simulink model "feed_lin_double_deriv_complete"  (R2022b)
settings: Solver=VariableStepAuto  StartTime=0.0  StopTime=15  RelTol=1e-3
model workspace (MAT data in the model file):
  initial_conditions = [0 0 0]
values from neighbouring files (symbols this model uses):
  initial_conditions_1 = [8, 8, 0]    [init.m]
  initial_conditions_2 = [6, 3, 2*pi]    [init.m]
  initial_conditions_3 = [-8, -8, 3*pi/2]    [init.m]
  initial_conditions_trans_2 = state_transformation([0,0,0], initial_conditions_2)    [init.m]
  initial_conditions_trans_3 = state_transformation([0,0,0], initial_conditions_3)    [init.m]
undefined symbols (not defined in the file or in its folder): initial_conditions_trans
settings Model: Creator=dipietrant  LastModifiedBy=Edp
settings SolverCC: AlgebraicLoopSolver=TrustRegion
settings DataIOCC: ReturnWorkspaceOutputs=off
settings DebuggingCC: UnconnectedInputMsg=warning  UnconnectedOutputMsg=warning  UnconnectedLineMsg=warning  SFMachineParentedDataDiag=warning
settings ModelReferenceCC: EnableRefExpFcnMdlSchedulingChecks=on
settings RTWCC: DLArmComputeVersion=19.05

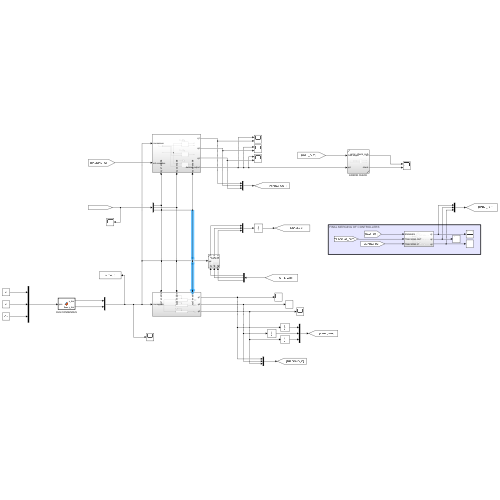
[thumbnail: Simulink's stored preview of the top-level diagram]
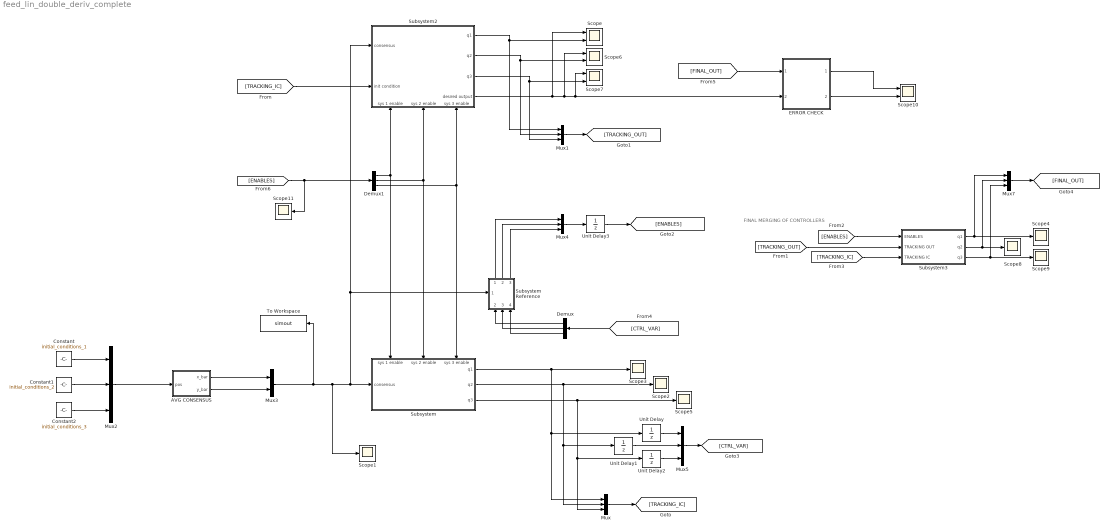
== system feed_lin_double_deriv_complete ==
  note: FINAL MERGING OF CONTROLLERS
  AVG CONSENSUS : MATLAB Function  TreatAsAtomicUnit=on
  Constant : Constant  Value=initial_conditions_1
  Constant1 : Constant  Value=initial_conditions_2
  Constant2 : Constant  Value=initial_conditions_3
  Demux : Demux  Outputs=3
  Demux1 : Demux  Outputs=3
  ERROR CHECK : Subsystem  ReferencedSubsystem=error_check_sub
  Mux{,1..2,4..5,7} (6 alike) : Mux  Inputs=3
  Mux3 : Mux  Inputs=2
  Scope{,6..7,10} (4 alike) : Scope  NumInputPorts=2
  Scope{1..5,8..9,11} (8 alike) : Scope
  Subsystem : Subsystem
      settings: PortSchema="{\"entries\":[{\"content\":{\"sides\":[{\"content\":{\"connectorIds\":[\"In1\"]},\"type\":\"ConnectorPlacement.EquallySpacedRectSide\",\"uuid\":\"b8325f4a-1506-42dc-8b3b-ec51295da985\"},{\"content\":{\"connectorIds\":[\"Out1\",\"Out2\",\"Out3\"],\"side\":\"RIGHT\"},\"type\":\"ConnectorPlacement.EquallySpacedRectSide\",\"uuid\":\"fb9dfe16-cc9c-4d6f-a089-d72d53b0d2ff\"},{\"content\":{\"connectorIds\":[\"In2\",\"In3\",\"In4\"],\"side\":\"TOP\"},\"type\":\"ConnectorPlacement.EquallySpacedRectSide\",\"uuid\":\"9b275e3a-3759-4fde-8298-bd376a2cee85\"}]},\"type\":\"ConnectorPlacement.EquallySpacedConnector\",\"uuid\":\"d20656d9-93c4-478d-bddd-a99c25c4725b\"}],\"packageUris\":[\"http://schema.mathworks.com/mf0/Connector/R2020b\"],\"version\":\"1.0\"}"
  Subsystem Reference : Subsystem  ReferencedSubsystem=controller_change
      settings: PortSchema="{\"entries\":[{\"content\":{\"sides\":[{\"content\":{\"connectorIds\":[\"In1\"]},\"type\":\"ConnectorPlacement.EquallySpacedRectSide\",\"uuid\":\"5cd3003d-d568-402f-bfb7-ab1f003474d5\"},{\"content\":{\"connectorIds\":[],\"side\":\"RIGHT\"},\"type\":\"ConnectorPlacement.EquallySpacedRectSide\",\"uuid\":\"2aacd520-5656-4ace-a561-d83f5de13db8\"},{\"content\":{\"connectorIds\":[\"Out1\",\"Out2\",\"Out3\"],\"side\":\"TOP\"},\"type\":\"ConnectorPlacement.EquallySpacedRectSide\",\"uuid\":\"c87f1391-dfec-417b-aa69-c1c2240fe0e2\"},{\"content\":{\"connectorIds\":[\"In2\",\"In3\",\"In4\"],\"side\":\"BOTTOM\"},\"type\":\"ConnectorPlacement.EquallySpacedRectSide\",\"uuid\":\"0817a7fd-038b-4a49-9ab5-3078e1b34ed6\"}]},\"type\":\"ConnectorPlacement.EquallySpacedConnector\",\"uuid\":\"1fba4bac-bef7-4725-afbb-950fb29d7a2b\"}],\"packageUris\":[\"http://schema.mathworks.com/mf0/Connector/R2020b\"],\"version\":\"1.0\"}"
  Subsystem2 : Subsystem
      settings: PortSchema="{\"entries\":[{\"content\":{\"sides\":[{\"content\":{\"connectorIds\":[\"In1\",\"In2\"]},\"type\":\"ConnectorPlacement.EquallySpacedRectSide\",\"uuid\":\"c7187f0f-6de3-44e8-9e0e-ba228c9cba05\"},{\"content\":{\"connectorIds\":[\"Out1\",\"Out2\",\"Out3\",\"Out4\"],\"side\":\"RIGHT\"},\"type\":\"ConnectorPlacement.EquallySpacedRectSide\",\"uuid\":\"09c5af45-e1de-4e92-aafe-d4959230805a\"},{\"content\":{\"connectorIds\":[],\"side\":\"TOP\"},\"type\":\"ConnectorPlacement.EquallySpacedRectSide\",\"uuid\":\"52f88a2b-e666-4633-98f7-6d0c847241cf\"},{\"content\":{\"connectorIds\":[\"In3\",\"In4\",\"In5\"],\"side\":\"BOTTOM\"},\"type\":\"ConnectorPlacement.EquallySpacedRectSide\",\"uuid\":\"0cb49b3b-0a2d-4d8e-878b-32676413b3c3\"}]},\"type\":\"ConnectorPlacement.EquallySpacedConnector\",\"uuid\":\"98e37247-887e-45d0-94e1-e2eafca9d3a3\"}],\"packageUris\":[\"http://schema.mathworks.com/mf0/Connector/R2020b\"],\"version\":\"1.0\"}"
  Subsystem3 : Subsystem
  To Workspace : ToWorkspace  VariableName=simout  SaveFormat=Structure With Time  SampleTime=-1
  Unit Delay : UnitDelay  InitialCondition=initial_conditions_1  SampleTime=-1  HasFrameUpgradeWarning=on
  Unit Delay1 : UnitDelay  InitialCondition=initial_conditions_2  SampleTime=-1  HasFrameUpgradeWarning=on
  Unit Delay2 : UnitDelay  InitialCondition=initial_conditions_3  SampleTime=-1  HasFrameUpgradeWarning=on
  Unit Delay3 : UnitDelay  InitialCondition=1  SampleTime=-1  HasFrameUpgradeWarning=on
  wires:
  Mux2/1 -> AVG CONSENSUS/1(pos)
  AVG CONSENSUS/1(x_bar) -> Mux3/1
  AVG CONSENSUS/2(y_bar) -> Mux3/2
  Constant1/1 -> Mux2/2
  Constant/1 -> Mux2/1
  Subsystem Reference/2 -> Mux4/2
  Constant2/1 -> Mux2/3
  Subsystem Reference/3 -> Mux4/3
  Subsystem Reference/1 -> Mux4/1
  Mux/1 -> [TRACKING_IC]
  [TRACKING_IC] -> Subsystem2/2(init condition)
  Subsystem2/1(q1) -> Mux1/1, Scope/2
  Subsystem2/2(q2) -> Mux1/2, Scope6/2
  Subsystem2/3(q3) -> Mux1/3, Scope7/2
  Mux1/1 -> [TRACKING_OUT]
  Mux4/1 -> Unit Delay3/1
  [ENABLES] -> Subsystem3/1(ENABLES)
  [TRACKING_OUT] -> Subsystem3/2(TRACKING OUT)
  [TRACKING_IC] -> Subsystem3/3(TRACKING IC)
  Mux3/1 -> To Workspace/1, Scope1/1, Subsystem Reference/1, Subsystem2/1(consensus), Subsystem/1(consensus)
  Unit Delay3/1 -> [ENABLES]
  Demux/3 -> Subsystem Reference/4
  Demux/2 -> Subsystem Reference/3
  Demux/1 -> Subsystem Reference/2
  [CTRL_VAR] -> Demux/1
  ERROR CHECK/2 -> Scope10/2
  ERROR CHECK/1 -> Scope10/1
  Subsystem2/4(desired output) -> Scope/1, Scope6/1, Scope7/1, ERROR CHECK/2
  [FINAL_OUT] -> ERROR CHECK/1
  Mux7/1 -> [FINAL_OUT]
  Subsystem3/3(q3) -> Mux7/3, Scope9/1
  Subsystem3/2(q2) -> Mux7/2, Scope8/1
  Subsystem3/1(q1) -> Mux7/1, Scope4/1
  Unit Delay2/1 -> Mux5/3
  Unit Delay1/1 -> Mux5/2
  Unit Delay/1 -> Mux5/1
  Mux5/1 -> [CTRL_VAR]
  Subsystem/3(q3) -> Scope5/1, Unit Delay2/1, Mux/3
  Subsystem/2(q2) -> Unit Delay1/1, Mux/2, Scope2/1
  Subsystem/1(q1) -> Unit Delay/1, Mux/1, Scope3/1
  Demux1/3 -> Subsystem/4(sys 3 enable), Subsystem2/5(sys 3 enable)
  Demux1/1 -> Subsystem/2(sys 1 enable), Subsystem2/3(sys 1 enable)
  Demux1/2 -> Subsystem/3(sys 2 enable), Subsystem2/4(sys 2 enable)
  [ENABLES] -> Demux1/1, Scope11/1

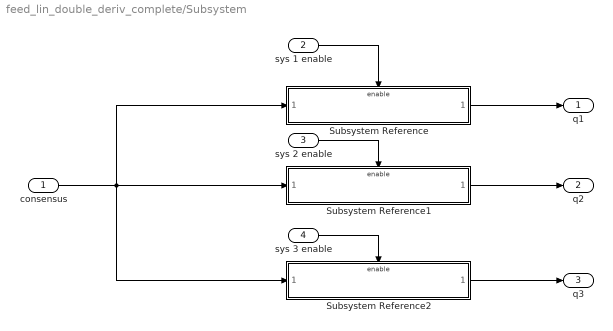
== system feed_lin_double_deriv_complete/Subsystem ==
  consensus : Inport
  sys 1 enable : Inport  Port=2
  sys 2 enable : Inport  Port=3
  sys 3 enable : Inport  Port=4
  Subsystem Reference : Subsystem  ReferencedSubsystem=posture_subsys  InitialCondition=initial_conditions_trans
  Subsystem Reference1 : Subsystem  ReferencedSubsystem=posture_subsys  InitialCondition=initial_conditions_trans_2
  Subsystem Reference2 : Subsystem  ReferencedSubsystem=posture_subsys  InitialCondition=initial_conditions_trans_3
  q1 : Outport
  q2 : Outport  Port=2
  q3 : Outport  Port=3
  wires:
  Subsystem Reference/1 -> q1/1
  Subsystem Reference1/1 -> q2/1
  consensus/1 -> Subsystem Reference1/1, Subsystem Reference2/1, Subsystem Reference/1
  sys 1 enable/1 -> Subsystem Reference/Enable
  sys 2 enable/1 -> Subsystem Reference1/Enable
  sys 3 enable/1 -> Subsystem Reference2/Enable
  Subsystem Reference2/1 -> q3/1

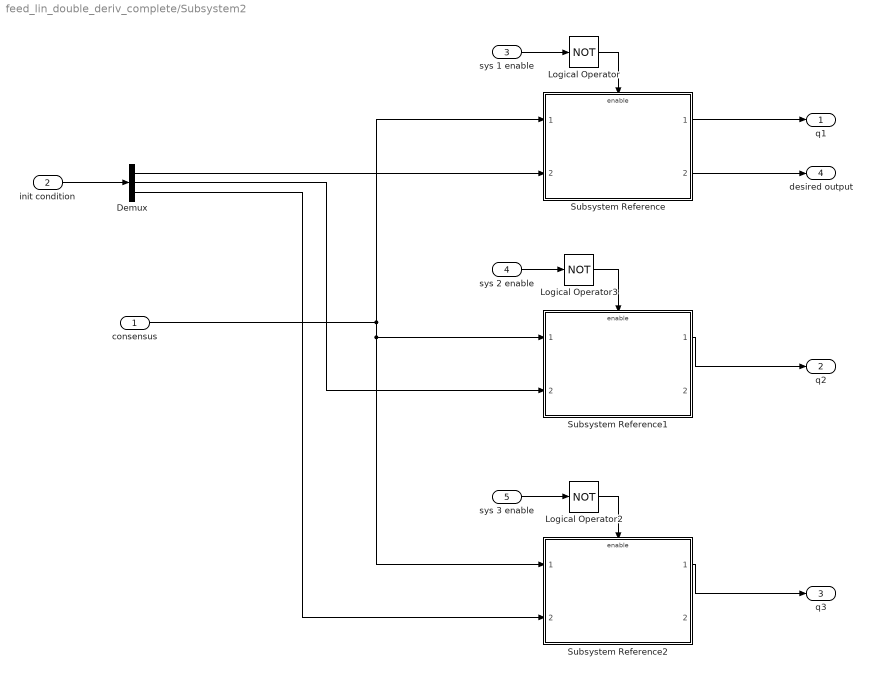
== system feed_lin_double_deriv_complete/Subsystem2 ==
  consensus : Inport
  init condition : Inport  Port=2
  sys 1 enable : Inport  Port=3
  sys 2 enable : Inport  Port=4
  sys 3 enable : Inport  Port=5
  Demux : Demux  Outputs=3
  Logical Operator : Logic  Operator=NOT  AllPortsSameDT=off  OutDataTypeStr=boolean
  Logical Operator2 : Logic  Operator=NOT  AllPortsSameDT=off  OutDataTypeStr=boolean
  Logical Operator3 : Logic  Operator=NOT  AllPortsSameDT=off  OutDataTypeStr=boolean
  Subsystem Reference : Subsystem  ReferencedSubsystem=feed_lin_double_deriv_sub
  Subsystem Reference1 : Subsystem  ReferencedSubsystem=feed_lin_double_deriv_sub
  Subsystem Reference2 : Subsystem  ReferencedSubsystem=feed_lin_double_deriv_sub
  q1 : Outport
  q2 : Outport  Port=2
  q3 : Outport  Port=3
  desired output : Outport  Port=4
  wires:
  sys 1 enable/1 -> Logical Operator/1
  Logical Operator/1 -> Subsystem Reference/Enable
  Subsystem Reference/1 -> q1/1
  sys 3 enable/1 -> Logical Operator2/1
  Logical Operator2/1 -> Subsystem Reference2/Enable
  Subsystem Reference1/1 -> q2/1
  Subsystem Reference2/1 -> q3/1
  consensus/1 -> Subsystem Reference2/1, Subsystem Reference1/1, Subsystem Reference/1
  init condition/1 -> Demux/1
  Demux/1 -> Subsystem Reference/2
  Demux/2 -> Subsystem Reference1/2
  Demux/3 -> Subsystem Reference2/2
  sys 2 enable/1 -> Logical Operator3/1
  Logical Operator3/1 -> Subsystem Reference1/Enable
  Subsystem Reference/2 -> desired output/1

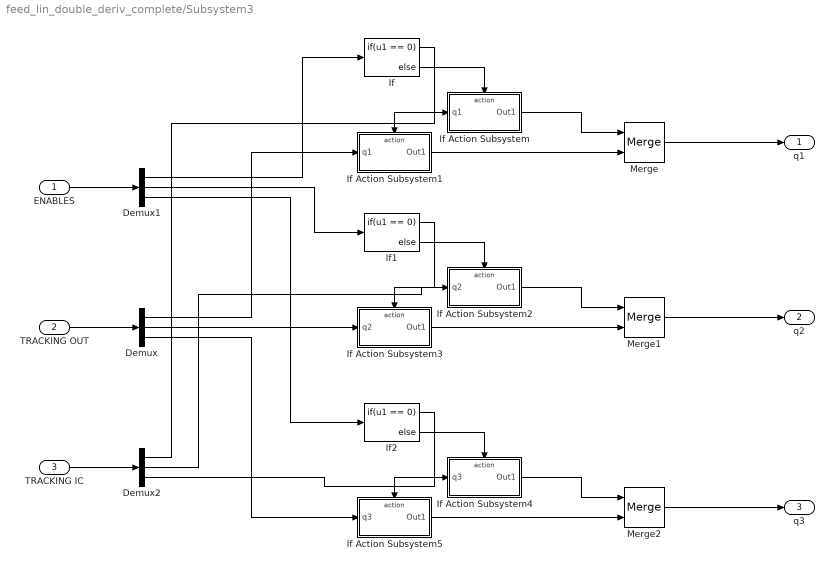
== system feed_lin_double_deriv_complete/Subsystem3 ==
  ENABLES : Inport
  TRACKING OUT : Inport  Port=2
  TRACKING IC : Inport  Port=3
  Demux : Demux  Outputs=3
  Demux1 : Demux  Outputs=3
  Demux2 : Demux  Outputs=3
  If : If  IfExpression=u1 == 0
  If Action Subsystem : Subsystem  TreatAsAtomicUnit=on
  If Action Subsystem1 : Subsystem  TreatAsAtomicUnit=on
  If Action Subsystem2 : Subsystem  TreatAsAtomicUnit=on
  If Action Subsystem3 : Subsystem  TreatAsAtomicUnit=on
  If Action Subsystem4 : Subsystem  TreatAsAtomicUnit=on
  If Action Subsystem5 : Subsystem  TreatAsAtomicUnit=on
  If1 : If  IfExpression=u1 == 0
  If2 : If  IfExpression=u1 == 0
  Merge : Merge
  Merge1 : Merge
  Merge2 : Merge
  q1 : Outport
  q2 : Outport  Port=2
  q3 : Outport  Port=3
  wires:
  Demux2/1 -> If Action Subsystem/1(q1)
  If Action Subsystem4/1(Out1) -> Merge2/1
  If1/1 -> If Action Subsystem3/Action
  If2/1 -> If Action Subsystem5/Action
  Demux/2 -> If Action Subsystem3/1(q2)
  If Action Subsystem5/1(Out1) -> Merge2/2
  Demux1/3 -> If2/1
  If2/2 -> If Action Subsystem4/Action
  Demux2/2 -> If Action Subsystem2/1(q2)
  If/2 -> If Action Subsystem/Action
  Demux/1 -> If Action Subsystem1/1(q1)
  Demux2/3 -> If Action Subsystem4/1(q3)
  Demux/3 -> If Action Subsystem5/1(q3)
  ENABLES/1 -> Demux1/1
  If/1 -> If Action Subsystem1/Action
  If Action Subsystem3/1(Out1) -> Merge1/2
  If Action Subsystem2/1(Out1) -> Merge1/1
  If1/2 -> If Action Subsystem2/Action
  Demux1/1 -> If/1
  If Action Subsystem1/1(Out1) -> Merge/2
  If Action Subsystem/1(Out1) -> Merge/1
  Demux1/2 -> If1/1
  TRACKING OUT/1 -> Demux/1
  Merge2/1 -> q3/1
  Merge/1 -> q1/1
  TRACKING IC/1 -> Demux2/1
  Merge1/1 -> q2/1

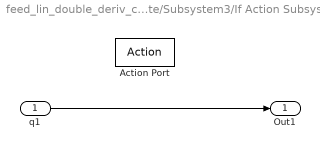
== system feed_lin_double_deriv_complete/Subsystem3/If Action Subsystem ==
  q1 : Inport
  Action Port : ActionPort  ActionPortLabel=else
  Out1 : Outport
  wires:
  q1/1 -> Out1/1

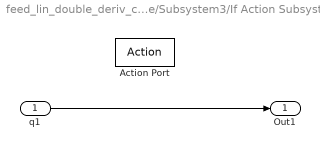
== system feed_lin_double_deriv_complete/Subsystem3/If Action Subsystem1 ==
  q1 : Inport
  Action Port : ActionPort  ActionPortLabel=if(u1 == 0)
  Out1 : Outport
  wires:
  q1/1 -> Out1/1

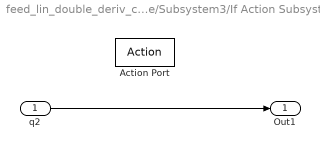
== system feed_lin_double_deriv_complete/Subsystem3/If Action Subsystem2 ==
  q2 : Inport
  Action Port : ActionPort  ActionPortLabel=else
  Out1 : Outport
  wires:
  q2/1 -> Out1/1

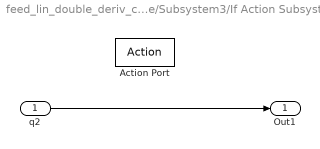
== system feed_lin_double_deriv_complete/Subsystem3/If Action Subsystem3 ==
  q2 : Inport
  Action Port : ActionPort  ActionPortLabel=if(u1 == 0)
  Out1 : Outport
  wires:
  q2/1 -> Out1/1

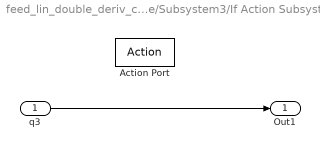
== system feed_lin_double_deriv_complete/Subsystem3/If Action Subsystem4 ==
  q3 : Inport
  Action Port : ActionPort  ActionPortLabel=else
  Out1 : Outport
  wires:
  q3/1 -> Out1/1

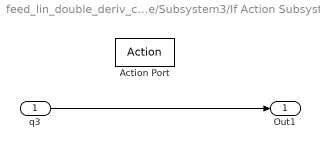
== system feed_lin_double_deriv_complete/Subsystem3/If Action Subsystem5 ==
  q3 : Inport
  Action Port : ActionPort  ActionPortLabel=if(u1 == 0)
  Out1 : Outport
  wires:
  q3/1 -> Out1/1

== matlab function feed_lin_double_deriv_complete/AVG CONSENSUS ==
  data: pos input; x_bar output; y_bar output
function [x_bar, y_bar] = fcn(pos)

x_bar = 0;
y_bar = 0;
n = 0;
for i=1:3:length(pos)
    x_bar = x_bar + pos(i);
    y_bar = y_bar + pos(i+1);
    n = n + 1; 
end 

x_bar = x_bar / n;
y_bar = y_bar / n;
